simulink model "lab10"  (Simulink 8.5)
settings: Solver=ode45  StartTime=0.0  StopTime=10000000  RelTol=1e-3
settings Model: Creator=Meteo  LastModifiedBy=Meteo
settings DataIOCC: SignalLoggingSaveFormat=Dataset
settings OptimizationCC: ExpressionDepthLimit=128
settings DebuggingCC: UnderspecifiedInitializationDetection=Simplified  MergeDetectMultiDrivingBlocksExec=error  FcnCallInpInsideContextMsg=EnableAllAsError  StateNameClashWarn=none
settings GRTTargetCC: CombineOutputUpdateFcns=on  GRTInterface=off

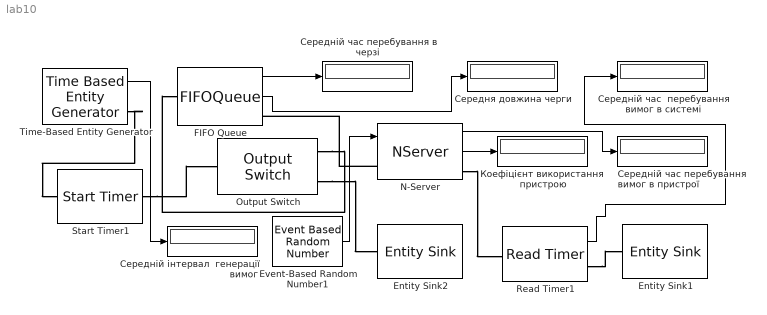
== system lab10 ==
  Entity Sink1 : EntitySink
  Entity Sink2 : EntitySink
  Event-Based Random Number1 : EventBasedRandomNumber  meanExp=17  Seed=61357
  FIFO Queue : FIFOQueue  Capacity=4  StatAverageWait=on  StatAverageQueueLength=on
      settings: OutputPortMap=o2,o3
  N-Server : NServer  NumberOfServers=2  ServiceTimeFrom=Signal port t  StatAverageWait=on  StatUtilization=on
      settings: OutputPortMap=o4,o5
  Output Switch : OutputSwitch  NumberOutputPorts=2
  Read Timer1 : ReadTimer  StatAverageTimeElapsed=on
      settings: OutputPortMap=o3
  Start Timer1 : StartTimer
  Time-Based Entity Generator : TimeBasedEntityGenerator  Distribution=Exponential  Period=27  InitialSeed=64574  Mean=27  StatAverageIntergenerationTime=on
      settings: OutputPortMap=o2
  Коефіцієнт використання  пристрою : Display
  Середня довжина черги : Display
  Середній час  перебування вимог в системі : Display
  "Середній час перебування  вимог в пристрої " : Display
  Середній час перебування в черзі : Display
  Середній інтервал  генерації вимог : Display
  wires:
  N-Server/1 -> "Середній час перебування  вимог в пристрої "/1
  Read Timer1/1 -> Середній час  перебування вимог в системі/1
  N-Server/2 -> Коефіцієнт використання  пристрою/1
  FIFO Queue/2 -> Середня довжина черги/1
  FIFO Queue/1 -> Середній час перебування в черзі/1
  Event-Based Random Number1/1 -> N-Server/1
  Time-Based Entity Generator/1 -> Середній інтервал  генерації вимог/1
  connections:
  N-Server/RConn1 -- Read Timer1/LConn1
  N-Server/LConn1 -- FIFO Queue/RConn1
  Start Timer1/RConn1 -- Output Switch/LConn1
  Read Timer1/RConn1 -- Entity Sink1/LConn1
  Time-Based Entity Generator/RConn1 -- Start Timer1/LConn1
  Output Switch/RConn1 -- FIFO Queue/LConn1
  Output Switch/RConn2 -- Entity Sink2/LConn1
